simulink model "ConfiguredVirtualVehicleModel"  (R2025b)
settings: Solver=ode14x  StartTime=0  StopTime=inf  FixedStep=.001  RelTol=1e-2  EnableMultiTasking=on
StopFcn:
  | %toc
undefined symbols (not defined in the file or in its folder): CtrlTcuInitGear, DriverPreviewDist, EnvAbsPrs, EnvAirTemp, EnvGrvty, EnvNomFrictionScaling, EnvNominalGrade, EnvWindVelX, EnvWindVelY, EnvWindVelZ, MotoFrmInert, MotoFrmLngth, MotoFrmMass, MotoLowrFrntFrkMass, MotoRearArmLngth, MotoRearArmMass, MotoUpprFrntFrkMass, PlntEngTqMax, RiderMass, Sim3dSensor, trackData
libraries: sm_lib x12, simulink x11, nesl_utility x8, sim3dgroundtruthsensorlib x2, autolibshared x2, vehdynlibdriver x2, instrumentseriallib x2, sharedtransform x1, vehdynlibviscommon x1, autolibutils x1, vehdynlibscenariocommon x1, vehdynlibsteering x1
(part 1 of 5)
settings Model: DataDictionary=VirtualMotoTemplate.sldd  ModifiedByFormat=The MathWorks, Inc.  PauseTimes=23.4  Creator=The MathWorks, Inc.  LastModifiedBy=The MathWorks, Inc.
settings SolverCC: ExtrapolationOrder=2.0  NumberNewtonIterations=2.0  DaesscMode=Fast  ZeroCrossAlgorithm=Adaptive  AlgebraicLoopSolver=TrustRegion  AutoInsertRateTranBlk=on  InsertRTBMode=Never (minimum delay)  DecoupledContinuousIntegration=on  MinimalZcImpactIntegration=on  MaxZcPerStep=1.0
settings DataIOCC: DSMLogging=off  ReturnWorkspaceOutputs=off
settings OptimizationCC: ReuseModelBlockBuffer=off
settings DebuggingCC: SignalInfNanChecking=error  ArtificialAlgebraicLoopMsg=none  MaskedZcDiagnostic=none  IgnoredZcDiagnostic=none  UnconnectedInputMsg=warning  UnconnectedOutputMsg=warning  UnconnectedLineMsg=warning  PregeneratedLibrarySubsystemCodeDiagnostic=none  SubsystemReferenceDiagnosticForUnitTest=warning  ArithmeticOperatorsInVariantConditions=warning
settings HardwareCC: UseEmbeddedCoderFeatures=off
settings ModelReferenceCC: EnableRefExpFcnMdlSchedulingChecks=on  ModelReferenceMinAlgLoopOccurrences=on  PropagateSignalLabelsOutOfModel=off
settings SFSimCC: SimUseLocalCustomCode=off
settings RTWCC: RTWUseLocalCustomCode=off  GPUComputeCapability=3.5  DLArmComputeVersion=19.05  LargeConstantGeneration=WriteOnlyDNNConstantsToDataFiles
settings ExplorerConfigSet: SimMechanicsOpenEditorOnUpdate=off  InternalSimMechanicsExplorerSettings="<ExplorerConfiguration><canonicalview>default</canonicalview><AnimationSetting><BasePlaybackSpeed>1.0</BasePlaybackSpeed><PlaybackSpeedFactor>0.5</PlaybackSpeedFactor></AnimationSetting><TilePanel><TileInfo><Tiles Columns=\"1\" Count=\"1\" Rows=\"1\"><Column Weight=\"1\"/><Row Weight=\"1\"/><Tile Height=\"1\" Width=\"1\" X=\"0\" Y=\"0\"/></Tiles></TileInfo><SceneInfo><SceneViewer><BGColor><R>0.60000002384185791</R><G>0.60000002384185791</G><B>0.60000002384185791</B></BGColor><Camera><DoPerspective>on</DoPerspective><Position><X>48.3730560002180638</X><Y>0.69720714407681017</Y><Z>1.00624025938607131</Z></Position><Center><X>47.6181790802191784</X><Y>1.35307362107727269</Y><Z>1.00624025938607131</Z></Center><Up><X>0</X><Y>0</Y><Z>1</Z></Up><ViewLimDist>1</ViewLimDist><YLim>0.466307658154998583</YLim><XLim>1.00155607891196818</XLim></Camera></SceneViewer></SceneInfo></TilePanel><MechEditorPanel><Cameras><Camera><Id>Camera1</Id><Value><Name>InplaneRightSide</Name><NativeCamera><PositionTrackingFeature>Motorcycle_Vehicle.Body_Steer_Suspension_Wheels.Body_Steer_Suspension_Wheels.In_Plane_Model.Chassis_Tires_and_Areo.Chassis_Body_Suspension_and_Steering.CHASSIS.Chassis_body.CPRr.Camera.Right.base.R</PositionTrackingFeature><CenterTrackingFeature>Motorcycle_Vehicle.Body_Steer_Suspension_Wheels.Body_Steer_Suspension_Wheels.In_Plane_Model.Chassis_Tires_and_Areo.Chassis_Body_Suspension_and_Steering.CHASSIS.Chassis_body.CPRr.Camera.Right.target.R</CenterTrackingFeature><UpVectorTrackingFeature>Motorcycle_Vehicle.Body_Steer_Suspension_Wheels.Body_Steer_Suspension_Wheels.In_Plane_Model.Chassis_Tires_and_Areo.Chassis_Body_Suspension_and_Steering.CHASSIS.Chassis_body.CPRr.Camera.Right.target.R</UpVectorTrackingFeature><CenterTrackingOrigin>off</CenterTrackingOrigin><CenterTrackingDirection>-Y</CenterTrackingDirection><UpVectorTrackingDirection>-Z</UpVectorTrackingDirection></NativeCamera></Value></Camera><Camera><Id>Camera2</Id><Value><Name>OutofPlaneRightSide</Name><NativeCamera><PositionTrackingFeature>Motorcycle_Vehicle.Body_Steer_Suspension_Wheels.Body_Steer_Suspension_Wheels.Out_of_Plane_Model.Chassis_Tires_and_Areo.Chassis_Body_Suspension_and_Steering.CHASSIS.Chassis_body.CPRr.Camera.Right.base.R</PositionTrackingFeature><CenterTrackingFeature>Motorcycle_Vehicle.Body_Steer_Suspension_Wheels.Body_Steer_Suspension_Wheels.Out_of_Plane_Model.Chassis_Tires_and_Areo.Chassis_Body_Suspension_and_Steering.CHASSIS.Chassis_body.CPRr.Camera.Right.base.R</CenterTrackingFeature><UpVectorTrackingFeature>Motorcycle_Vehicle.Body_Steer_Suspension_Wheels.Body_Steer_Suspension_Wheels.Out_of_Plane_Model.Chassis_Tires_and_Areo.Chassis_Body_Suspension_and_Steering.CHASSIS.Chassis_body.CPRr.Camera.Right.base.R</UpVectorTrackingFeature><CenterTrackingOrigin>off</CenterTrackingOrigin><CenterTrackingDirection>-Y</CenterTrackingDirection><UpVectorTrackingDirection>-Z</UpVectorTrackingDirection></NativeCamera></Value></Camera></Cameras><GfxPanelCameraMap><MapElement CameraMLId=\"Camera2\" GfxPanelIndex=\"0\"/></GfxPanelCameraMap><VideoCreator><PlaybackSpeedRatio>1.0</PlaybackSpeedRatio><FrameRate>30</FrameRate><VideoFormat>Motion JPEG AVI</VideoFormat><FrameSize>auto</FrameSize></VideoCreator></MechEditorPanel></ExplorerConfiguration>"

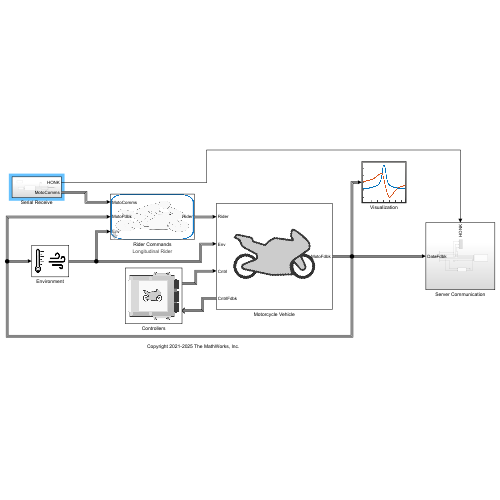
[thumbnail: Simulink's stored preview of the top-level diagram]
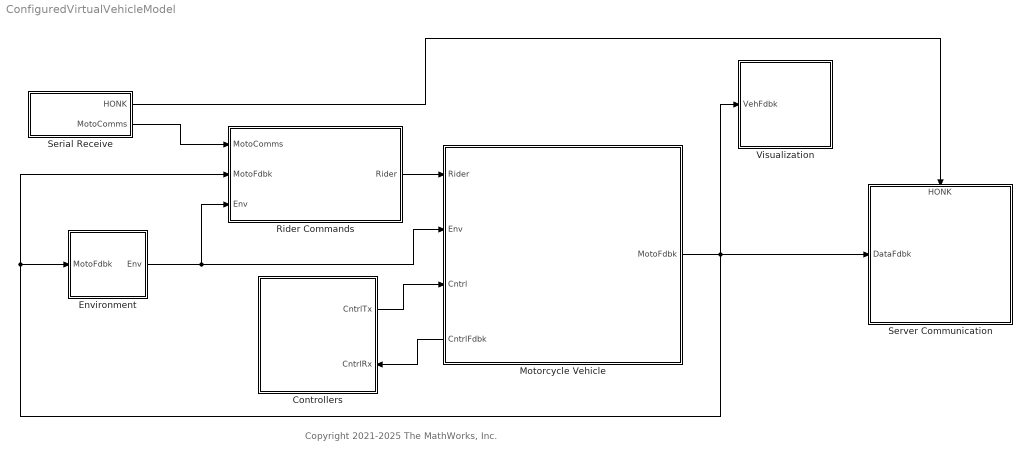
== system ConfiguredVirtualVehicleModel ==
  note: Copyright 2021-2025 The MathWorks, Inc.
  Controllers : Subsystem
      settings: PortSchema="{\"entries\":[{\"content\":{\"sides\":[{\"content\":{},\"type\":\"ConnectorPlacement.EquallySpacedRectSide\",\"uuid\":\"d3abfdf3-59f3-4762-8e4e-957745a11e2c\"},{\"content\":{\"connectorIds\":[\"Out1\",\"In1\"],\"side\":\"RIGHT\"},\"type\":\"ConnectorPlacement.EquallySpacedRectSide\",\"uuid\":\"4c115717-9c17-4631-bd95-1f831e7f83d7\"},{\"content\":{\"side\":\"TOP\"},\"type\":\"ConnectorPlacement.EquallySpacedRectSide\",\"uuid\":\"d2ccb451-5fc1-4147-9a0c-1582624fa182\"}]},\"type\":\"ConnectorPlacement.EquallySpacedConnector\",\"uuid\":\"cab9e2c1-ce8a-4f9c-a024-cef64f8d49c6\"}],\"packageUris\":[\"http://schema.mathworks.com/mf0/Connector/R2020b\"],\"version\":\"1.0\"}"
      mask Display: image('motoECU.png')
  Environment : Subsystem
      mask Display: image('Enviroment.png')
  Motorcycle Vehicle : Subsystem
      settings: PortSchema="{\"entries\":[{\"content\":{\"sides\":[{\"content\":{\"connectorIds\":[\"In1\",\"In2\",\"In3\",\"Out2\"]},\"type\":\"ConnectorPlacement.EquallySpacedRectSide\",\"uuid\":\"175d7041-2aff-4cd5-b9c0-3998d48105ea\"},{\"content\":{\"connectorIds\":[\"Out1\"],\"side\":\"RIGHT\"},\"type\":\"ConnectorPlacement.EquallySpacedRectSide\",\"uuid\":\"0f698ea4-f06f-4552-98b1-af1f0960853e\"},{\"content\":{\"side\":\"TOP\"},\"type\":\"ConnectorPlacement.EquallySpacedRectSide\",\"uuid\":\"8127d405-6a03-4548-a956-3e3bb7246319\"}]},\"type\":\"ConnectorPlacement.EquallySpacedConnector\",\"uuid\":\"b217a386-2802-4b5f-8626-423e606b91b2\"}],\"packageUris\":[\"http://schema.mathworks.com/mf0/Connector/R2020b\"],\"version\":\"1.0\"}"
      mask Display: image('moto.png')
  Rider Commands : Subsystem  VariantControl=0  mask{driverType=Longitudinal Rider, TorqueControlType=No torque control, A=0, D=0.1, I=5, P=150, OutSatLowLmt=-100, OutSatUpLmt=100}
      mask prompts: driverType "Rider type"; TorqueControlType "Torque control"; A "vdynblks:vehdynSteeringSystem:blkPrm_AntiwindGain"; D "vdynblks:vehdynSteeringSystem:blkPrm_DGain"; I "vdynblks:vehdynSteeringSystem:blkPrm_IGain"; P "vdynblks:vehdynSteeringSystem:blkPrm_PGain"; OutSatLowLmt "vdynblks:vehdynSteeringSystem:blkPrm_OutSatLowLmt"; OutSatUpLmt "vdynblks:vehdynSteeringSystem:blkPrm_OutSatUpLmt"
      mask init:
      | [~]=vdynblksdrvrconfig(gcb);
      settings: AttributesFormatString=%<driverType>
      mask Help: eval('vdynblkshelp(''vdmtrrider'')');
      mask TypeOptions driverType: Longitudinal Rider | Open Loop
      mask Callback driverType: [~]=vdynblksdrvrconfig(gcb);
      mask TypeOptions TorqueControlType: Torque PID control | No torque control | Look ahead point model | PID Control
      mask DialogControl A Prompt: Integral anti-windup gain, A []:
      mask DialogControl D Prompt: Derivative gain, D []:
      mask DialogControl I Prompt: Integral gain, I []:
      mask DialogControl P Prompt: Proportional gain, P []:
      mask DialogControl OutSatLowLmt Prompt: Steering torque output saturation lower limit, OutSatLowLmt [Nm]:
      mask DialogControl OutSatUpLmt Prompt: Steering torque output saturation upper limit, OutSatUpLmt [Nm]:
      mask Display: image('rider.png'); % Use "Edit Image" on toolstrip to change.
  Serial Receive : Subsystem
  Server Communication : Subsystem
      settings: PortSchema="{\"entries\":[{\"content\":{\"sides\":[{\"content\":{\"connectorIds\":[\"In1\"]},\"type\":\"ConnectorPlacement.EquallySpacedRectSide\",\"uuid\":\"07e3cf90-2a4b-4b6a-90e3-ec137f6b52d9\"},{\"content\":{\"side\":\"RIGHT\"},\"type\":\"ConnectorPlacement.EquallySpacedRectSide\",\"uuid\":\"79c66d88-e2e2-4982-8f08-c82342e6913b\"},{\"content\":{\"connectorIds\":[\"In2\"],\"side\":\"TOP\"},\"type\":\"ConnectorPlacement.EquallySpacedRectSide\",\"uuid\":\"449d2507-f600-4b7d-af9b-b4af7bc07d5d\"}]},\"type\":\"ConnectorPlacement.EquallySpacedConnector\",\"uuid\":\"5f8e3617-5497-45d3-8aaf-8e2d249ba135\"}],\"packageUris\":[\"http://schema.mathworks.com/mf0/Connector/R2020b\"],\"version\":\"1.0\"}"
  Visualization : Subsystem
      mask Display: image('Visualization.png')
  wires:
  Controllers/1(CntrlTx) -> Motorcycle Vehicle/3(Cntrl)
  Motorcycle Vehicle/2(CntrlFdbk) -> Controllers/1(CntrlRx)
  Environment/1(Env) -> Rider Commands/3(Env), Motorcycle Vehicle/2(Env)
  Motorcycle Vehicle/1(MotoFdbk) -> Server Communication/1(DataFdbk), Rider Commands/2(MotoFdbk), Environment/1(MotoFdbk), Visualization/1(VehFdbk)
  Rider Commands/1(Rider) -> Motorcycle Vehicle/1(Rider)
  Serial Receive/2(MotoComms) -> Rider Commands/1(MotoComms)
  Serial Receive/1(HONK) -> Server Communication/2(HONK)

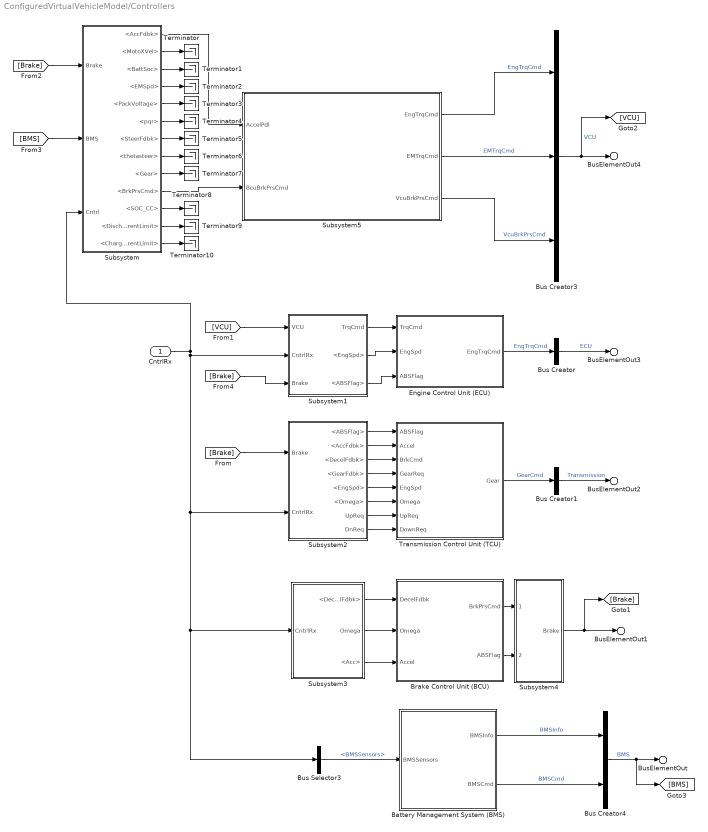
== system ConfiguredVirtualVehicleModel/Controllers ==
  CntrlRx : Inport
  Battery Management System (BMS) : Subsystem  Variant=on  VariantControlMode=label  LabelModeActiveChoice=NoBMS
  Brake Control Unit (BCU) : Subsystem  Variant=on  VariantChoicesSpecifier={'OpenLoopController'}  VariantControlMode=label  LabelModeActiveChoice=OpenLoopController
  Bus Creator : BusCreator  Inputs=1
  Bus Creator1 : BusCreator  Inputs=1
  Bus Creator3 : BusCreator  Inputs=3
  Bus Creator4 : BusCreator  Inputs=2
  Bus Selector3 : BusSelector  OutputSignals=Battery.BMSSensors
  Engine Control Unit (ECU) : Subsystem  Variant=on  VariantChoicesSpecifier={'MotoSimpleECU'}  VariantControlMode=label  LabelModeActiveChoice=MotoSimpleECU
  Subsystem : Subsystem
  Subsystem1 : Subsystem
  Subsystem2 : Subsystem
  Subsystem3 : Subsystem
  Subsystem4 : Subsystem
  Subsystem5 : Subsystem
  Terminator{,1..10} (11 alike) : Terminator
  Transmission Control Unit (TCU) : Subsystem  Variant=on  VariantChoicesSpecifier={'RiderPassThrough'}  VariantControlMode=label  VariantControl=Variant1  LabelModeActiveChoice=RiderPassThrough
  BusElementOut : Outport  PortName=CntrlTx  Element=BMS
  BusElementOut1 : Outport  PortName=CntrlTx  Element=Brake
  BusElementOut2 : Outport  PortName=CntrlTx  Element=Transmission
  BusElementOut3 : Outport  PortName=CntrlTx  Element=ECU
  BusElementOut4 : Outport  PortName=CntrlTx  Element=VCU
  wires:
  Bus Creator/1 -> BusElementOut3/1  "ECU"
  Bus Creator1/1 -> BusElementOut2/1  "Transmission"
  Engine Control Unit (ECU)/1(EngTrqCmd) -> Bus Creator/1  "EngTrqCmd"
  Transmission Control Unit (TCU)/1(" Gear") -> Bus Creator1/1  "GearCmd"
  CntrlRx/1 -> Subsystem1/2(CntrlRx), Subsystem3/1(CntrlRx), Bus Selector3/1, Subsystem2/2(CntrlRx), Subsystem/3(Cntrl)
  Bus Selector3/1 -> Battery Management System (BMS)/1(BMSSensors)  "<BMSSensors>"
  Battery Management System (BMS)/2(BMSCmd) -> Bus Creator4/2  "BMSCmd"
  Bus Creator4/1 -> [BMS], BusElementOut/1  "BMS"
  Battery Management System (BMS)/1(BMSInfo) -> Bus Creator4/1  "BMSInfo"
  Bus Creator3/1 -> [VCU], BusElementOut4/1  "VCU"
  Subsystem5/1(EngTrqCmd) -> Bus Creator3/1  "EngTrqCmd"
  Subsystem5/2(EMTrqCmd) -> Bus Creator3/2  "EMTrqCmd"
  Subsystem5/3(VcuBrkPrsCmd) -> Bus Creator3/3  "VcuBrkPrsCmd"
  [Brake] -> Subsystem/1(Brake)
  [BMS] -> Subsystem/2(BMS)
  Subsystem/1(<AccFdbk>) -> Subsystem5/1(AccelPdl)
  Subsystem/10(<BrkPrsCmd>) -> Subsystem5/2(BcuBrkPrsCmd)
  [Brake] -> Subsystem1/3(Brake)
  Subsystem1/2(<EngSpd>) -> Engine Control Unit (ECU)/2(EngSpd)
  Subsystem1/3(<ABSFlag>) -> Engine Control Unit (ECU)/3(ABSFlag)
  [Brake] -> Subsystem2/1(Brake)
  Subsystem2/1(<ABSFlag>) -> Transmission Control Unit (TCU)/1(ABSFlag)
  Subsystem2/2(<AccFdbk>) -> Transmission Control Unit (TCU)/2(Accel)
  Subsystem2/3(<DecelFdbk>) -> Transmission Control Unit (TCU)/3(BrkCmd)
  Subsystem2/4(<GearFdbk>) -> Transmission Control Unit (TCU)/4(GearReq)
  Subsystem2/5(<EngSpd>) -> Transmission Control Unit (TCU)/5(EngSpd)
  Subsystem2/6(<Omega>) -> Transmission Control Unit (TCU)/6(Omega)
  Subsystem3/1(<DecelFdbk>) -> Brake Control Unit (BCU)/1(DecelFdbk)
  Subsystem3/2(Omega) -> Brake Control Unit (BCU)/2(Omega)
  Subsystem3/3(<Acc>) -> Brake Control Unit (BCU)/3(Accel)
  Subsystem2/7(UpReq) -> Transmission Control Unit (TCU)/7(UpReq)
  Subsystem2/8(DnReq) -> Transmission Control Unit (TCU)/8(DownReq)
  Subsystem4/1(Brake) -> [Brake], BusElementOut1/1
  Brake Control Unit (BCU)/1(BrkPrsCmd) -> Subsystem4/1(BrkPrsCmd)
  Brake Control Unit (BCU)/2(ABSFlag) -> Subsystem4/2(ABSFlag)
  Subsystem/2(<MotoXVel>) -> Terminator/1
  Subsystem/3(<BattSoc>) -> Terminator1/1
  Subsystem/4(<EMSpd>) -> Terminator2/1
  Subsystem/5(<PackVoltage>) -> Terminator3/1
  Subsystem/6(<pqr>) -> Terminator4/1
  Subsystem/7(<SteerFdbk>) -> Terminator5/1
  Subsystem/8(<thetasteer>) -> Terminator6/1
  Subsystem/9(<Gear>) -> Terminator7/1
  Subsystem/11(<SOC_CC>) -> Terminator8/1
  Subsystem/12(<DischargeCurrentLimit>) -> Terminator9/1
  Subsystem/13(<ChargeCurrentLimit>) -> Terminator10/1
  [VCU] -> Subsystem1/1(VCU)
  Subsystem1/1(TrqCmd) -> Engine Control Unit (ECU)/1(TrqCmd)

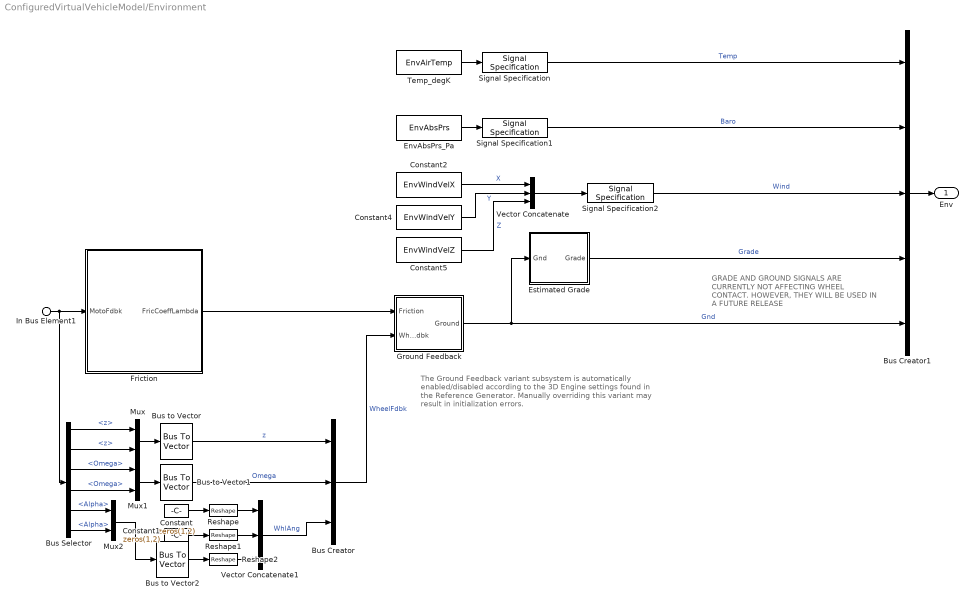
== system ConfiguredVirtualVehicleModel/Environment ==
  note: GRADE AND GROUND SIGNALS ARE CURRENTLY NOT AFFECTING WHEEL CONTACT. HOWEVER, THEY WILL BE USED IN A FUTURE RELEASE
  note: The Ground Feedback variant subsystem is automatically enabled/disabled according to the 3D Engine settings found in the Reference Generator.
      | Manually overriding this variant may result in initialization errors.
  In Bus Element1 : Inport  PortName=MotoFdbk
  Bus Creator : BusCreator  Inputs=3
  Bus Creator1 : BusCreator  Inputs=5
  Bus Selector : BusSelector  OutputSignals=Whl.Genrl.Frnt.Cp.Disp.z,Whl.Genrl.Rear.Cp.Disp.z,Wheels.FrontTire.Omega,Wheels.RearTire.Omega,Wheels.FrontTire.Alpha,Wheels.RearTire.Alpha
  Bus to Vector : BusToVector
  Bus to Vector1 : BusToVector
  Bus to Vector2 : BusToVector
  Constant : Constant  Value=zeros(1,2)
  Constant1 : Constant  Value=zeros(1,2)
  Constant2 : Constant  Value=EnvWindVelX  SampleTime=0
  Constant4 : Constant  Value=EnvWindVelY  SampleTime=0
  Constant5 : Constant  Value=EnvWindVelZ  SampleTime=0
  EnvAbsPrs_Pa : Constant  Value=EnvAbsPrs  SampleTime=0
  Estimated Grade : Subsystem
  Friction : Subsystem  Variant=on  VariantControlMode=label  VariantControl=Choice  LabelModeActiveChoice=Constant Friction
  Ground Feedback : Subsystem  Variant=on  VariantControlMode=label  LabelModeActiveChoice=0
  Mux : Mux  Inputs=2
  Mux1 : Mux  Inputs=2
  Mux2 : Mux  Inputs=2
  Reshape : Reshape  OutputDimensionality=Row vector (2-D)
  Reshape1 : Reshape  OutputDimensionality=Row vector (2-D)
  Reshape2 : Reshape  OutputDimensionality=Row vector (2-D)
  Signal Specification : SignalSpecification  Unit=K
  Signal Specification1 : SignalSpecification  Unit=Pa
  Signal Specification2 : SignalSpecification  Unit=m/s
  Temp_degK : Constant  Value=EnvAirTemp  SampleTime=0
  Vector Concatenate : Concatenate  NumInputs=3
  Vector Concatenate1 : Concatenate  NumInputs=3  Mode=Multidimensional array
  Env : Outport  VectorParamsAs1DForOutWhenUnconnected=off
  wires:
  Constant5/1 -> Vector Concatenate/3  "Z"
  Signal Specification2/1 -> Bus Creator1/3  "Wind"
  Constant4/1 -> Vector Concatenate/2  "Y"
  Ground Feedback/1(Ground) -> Bus Creator1/5, Estimated Grade/1(Gnd)  "Gnd"
  Bus Creator1/1 -> Env/1
  Signal Specification/1 -> Bus Creator1/1  "Temp"
  Signal Specification1/1 -> Bus Creator1/2  "Baro"
  Friction/1(FricCoeffLambda) -> Ground Feedback/1(Friction)
  Estimated Grade/1(Grade) -> Bus Creator1/4  "Grade"
  In Bus Element1/1 -> Friction/1(MotoFdbk), Bus Selector/1
  Bus Selector/2 -> Mux/2  "<z>"
  Bus Selector/1 -> Mux/1  "<z>"
  Mux/1 -> Bus to Vector/1
  Bus to Vector/1 -> Bus Creator/1  "z"
  Bus Selector/3 -> Mux1/1  "<Omega>"
  Bus Selector/4 -> Mux1/2  "<Omega>"
  Mux1/1 -> Bus to Vector1/1
  Bus to Vector1/1 -> Bus Creator/2  "Omega"
  Bus Selector/5 -> Mux2/1  "<Alpha>"
  Bus Selector/6 -> Mux2/2  "<Alpha>"
  Mux2/1 -> Bus to Vector2/1
  Constant/1 -> Reshape/1
  Constant1/1 -> Reshape1/1
  Bus to Vector2/1 -> Reshape2/1
  Reshape/1 -> Vector Concatenate1/1
  Reshape1/1 -> Vector Concatenate1/2
  Reshape2/1 -> Vector Concatenate1/3
  Vector Concatenate1/1 -> Bus Creator/3  "WhlAng"
  Bus Creator/1 -> Ground Feedback/2(WheelFdbk)  "WheelFdbk"
  Constant2/1 -> Vector Concatenate/1  "X"
  Temp_degK/1 -> Signal Specification/1
  EnvAbsPrs_Pa/1 -> Signal Specification1/1
  Vector Concatenate/1 -> Signal Specification2/1

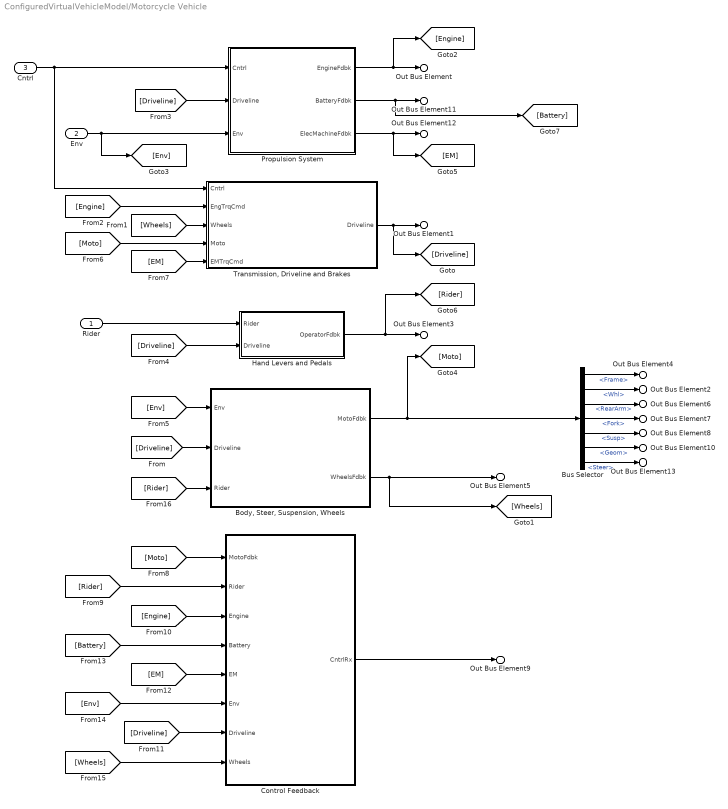
== system ConfiguredVirtualVehicleModel/Motorcycle Vehicle ==
  Rider : Inport
  Env : Inport  Port=2
  Cntrl : Inport  Port=3
  "Body, Steer, Suspension, Wheels" : Subsystem
      mask Display: image('$imagefile'); % Use "Edit Image" on toolstrip to change.
  Bus Selector : BusSelector  OutputSignals=Frame,Whl,RearArm,Fork,Susp,Geom,Steer
  Control Feedback : Subsystem
  Hand Levers and Pedals : Subsystem
  Propulsion System : Subsystem
      mask Display: image('$imagefile'); % Use "Edit Image" on toolstrip to change.
  "Transmission, Driveline and Brakes" : Subsystem
      mask Display: image('$imagefile'); % Use "Edit Image" on toolstrip to change.
  Out Bus Element : Outport  PortName=MotoFdbk  Element=Engine
  Out Bus Element3 : Outport  PortName=MotoFdbk  Element=Rider
  Out Bus Element4 : Outport  PortName=MotoFdbk  Element=Body
  Out Bus Element5 : Outport  PortName=MotoFdbk  Element=Wheels
  Out Bus Element1 : Outport  PortName=MotoFdbk  Element=Driveline
  Out Bus Element2 : Outport  PortName=MotoFdbk  Element=Whl
  Out Bus Element6 : Outport  PortName=MotoFdbk  Element=RearArm
  Out Bus Element7 : Outport  PortName=MotoFdbk  Element=Fork
  Out Bus Element8 : Outport  PortName=MotoFdbk  Element=Susp
  Out Bus Element10 : Outport  PortName=MotoFdbk  Element=Geom
  Out Bus Element11 : Outport  PortName=MotoFdbk  Element=Battery
  Out Bus Element12 : Outport  PortName=MotoFdbk  Element=ElecMachine
  Out Bus Element13 : Outport  PortName=MotoFdbk  Element=Steer
  Out Bus Element9 : Outport  Port=2  PortName=CntrlFdbk
  wires:
  Bus Selector/1 -> Out Bus Element4/1  "<Frame>"
  Bus Selector/2 -> Out Bus Element2/1  "<Whl>"
  Bus Selector/3 -> Out Bus Element6/1  "<RearArm>"
  Bus Selector/4 -> Out Bus Element7/1  "<Fork>"
  Bus Selector/5 -> Out Bus Element8/1  "<Susp>"
  Bus Selector/6 -> Out Bus Element10/1  "<Geom>"
  Propulsion System/1(EngineFdbk) -> [Engine], Out Bus Element/1
  [Driveline] -> Propulsion System/2(Driveline)
  "Transmission, Driveline and Brakes"/1(Driveline) -> [Driveline], Out Bus Element1/1
  [Engine] -> "Transmission, Driveline and Brakes"/2(EngTrqCmd)
  [Wheels] -> "Transmission, Driveline and Brakes"/3(Wheels)
  [Moto] -> "Transmission, Driveline and Brakes"/4(Moto)
  Propulsion System/2(BatteryFdbk) -> [Battery], Out Bus Element11/1
  Propulsion System/3(ElecMachineFdbk) -> Out Bus Element12/1, [EM]
  Rider/1 -> Hand Levers and Pedals/1(Rider)
  [Driveline] -> Hand Levers and Pedals/2(Driveline)
  Hand Levers and Pedals/1(OperatorFdbk) -> [Rider], Out Bus Element3/1
  "Body, Steer, Suspension, Wheels"/1(MotoFdbk) -> Bus Selector/1, [Moto]
  "Body, Steer, Suspension, Wheels"/2(WheelsFdbk) -> [Wheels], Out Bus Element5/1
  [Driveline] -> "Body, Steer, Suspension, Wheels"/2(Driveline)
  Env/1 -> [Env], Propulsion System/3(Env)
  [Env] -> "Body, Steer, Suspension, Wheels"/1(Env)
  [EM] -> "Transmission, Driveline and Brakes"/5(EMTrqCmd)
  Cntrl/1 -> "Transmission, Driveline and Brakes"/1(Cntrl), Propulsion System/1(Cntrl)
  Control Feedback/1(CntrlRx) -> Out Bus Element9/1
  [Moto] -> Control Feedback/1(MotoFdbk)
  [Rider] -> Control Feedback/2(Rider)
  [Engine] -> Control Feedback/3(Engine)
  [EM] -> Control Feedback/5(EM)
  [Battery] -> Control Feedback/4(Battery)
  [Driveline] -> Control Feedback/7(Driveline)
  [Env] -> Control Feedback/6(Env)
  [Wheels] -> Control Feedback/8(Wheels)
  [Rider] -> "Body, Steer, Suspension, Wheels"/3(Rider)
  Bus Selector/7 -> Out Bus Element13/1  "<Steer>"

== system ConfiguredVirtualVehicleModel/Rider Commands ==
  MotoComms : Inport
  MotoFdbk : Inport  Port=2
  Env : Inport  Port=3
  GearGround : Ground
  Rider Commands : Subsystem  Variant=on  VariantControl=Variant1
  Torque Control : Subsystem  Variant=on
  Rider : Outport  VectorParamsAs1DForOutWhenUnconnected=off
  wires:
  MotoComms/1 -> Torque Control/1(MotoRef), Rider Commands/1(MotoComms)
  MotoFdbk/1 -> Torque Control/2(MotoFdbk), Rider Commands/2(MotoFdbk)
  Rider Commands/1(" Rider") -> Torque Control/3(RiderInput)
  Env/1 -> Rider Commands/3(Env)
  Torque Control/1(Rider) -> Rider/1
  GearGround/1 -> Rider Commands/4(GearCmd)

== system ConfiguredVirtualVehicleModel/Serial Receive ==
  Bus Creator : BusCreator  Inputs=3
  Decode : MATLAB Function  TreatAsAtomicUnit=on
  RT : RateTransition  Deterministic=off  OutPortSampleTime=0.001
  Scope : Scope
      settings: ActiveDisplayYMinimum=0.59365579475349917  ActiveDisplayYMaximum=0.83764180505363828  DataLoggingVariableName=ScopeData3
  Serial Configuration : instrumentseriallib/Serial Configuration  Priority=-200000  PortSel=COM6  Port=COM6  ComPort=COM6  BaudRate=115200  DataBits=8  Parity=none  StopBits=1  ByteOrder=little-endian  FlowControl=none  Timeout=10  SimulateUsing=Interpreted execution  BlockInModel=on  aMode=1
  Serial Receive : instrumentseriallib/Serial Receive  Priority=1  PortSel=COM6  Port=COM6  ComPort=COM6  DataType=uint8  SaveDataType=uint8  ToggleHeader=off  Header=[]  ToggleDataSize=on  DataSize=[1 1]  ToggleTerminator=off  Terminator=<none>  CustomTerminator=[]  InputFormat=Column major  EnableBlockingMode=on  ActionDataUnavailable=Output last received value  ActionWhenDataUnavailable=Output last received value  CustomValue=0  SampleTime=0.01  SimulateUsing=Interpreted execution  BlockInModel=on  aMode=1  LibraryInUse=instrumentlib
  HONK : Outport
  MotoComms : Outport  Port=2
  wires:
  Serial Receive/1 -> Decode/1(rawByte)
  Bus Creator/1 -> MotoComms/1  "MotoComms"
  RT/1 -> HONK/1
  Decode/1(Accel) -> Scope/1, Bus Creator/1  "Accel"
  Decode/2(Decel) -> Bus Creator/2  "Decel"
  Decode/3(Gear) -> Bus Creator/3  "Gear"
  Decode/4(HONK) -> RT/1  "Decel"

== system ConfiguredVirtualVehicleModel/Server Communication ==
  DataFdbk : Inport
  HONK : Inport  Port=2
  Bus Selector : BusSelector  OutputSignals=Wheels.RearTire.Omega,Engine.EngineInfo.ExhManGasTemp,Engine.EngineInfo.EoCO2,Engine.EngineInfo.EngSpd,Engine.EngineInfo.FuelVolFlw,Body.BdyFrm.Cg.Vel.xdot
  Performance Calculations : Subsystem
  "Steer, Velocity, Lat Accel" : Scope  NumInputPorts=3
      settings: ActiveDisplayYMinimum=-569.38084213892614  ActiveDisplayYMaximum=94.564320801759081  DataLoggingVariableName=ScopeData2
  Terminator1 : Terminator
  UDPSend : MATLAB Function  TreatAsAtomicUnit=on
  wires:
  DataFdbk/1 -> Bus Selector/1
  Bus Selector/1 -> "Steer, Velocity, Lat Accel"/1, UDPSend/2(angspeed)  "<Omega>"
  Bus Selector/2 -> UDPSend/3(temp), "Steer, Velocity, Lat Accel"/3  "<ExhManGasTemp>"
  Bus Selector/3 -> UDPSend/4(emissions)  "<EoCO2>"
  Bus Selector/4 -> "Steer, Velocity, Lat Accel"/2, UDPSend/1(engspeed)  "<EngSpd>"
  HONK/1 -> UDPSend/6(HONK)
  Performance Calculations/1(US MPG) -> Terminator1/1
  Bus Selector/6 -> Performance Calculations/1(VehSpd)  "<xdot>"
  Bus Selector/5 -> Performance Calculations/2(FuelVolFlow)  "<FuelVolFlw>"
  Performance Calculations/2(L/100Km) -> UDPSend/5(fuel)

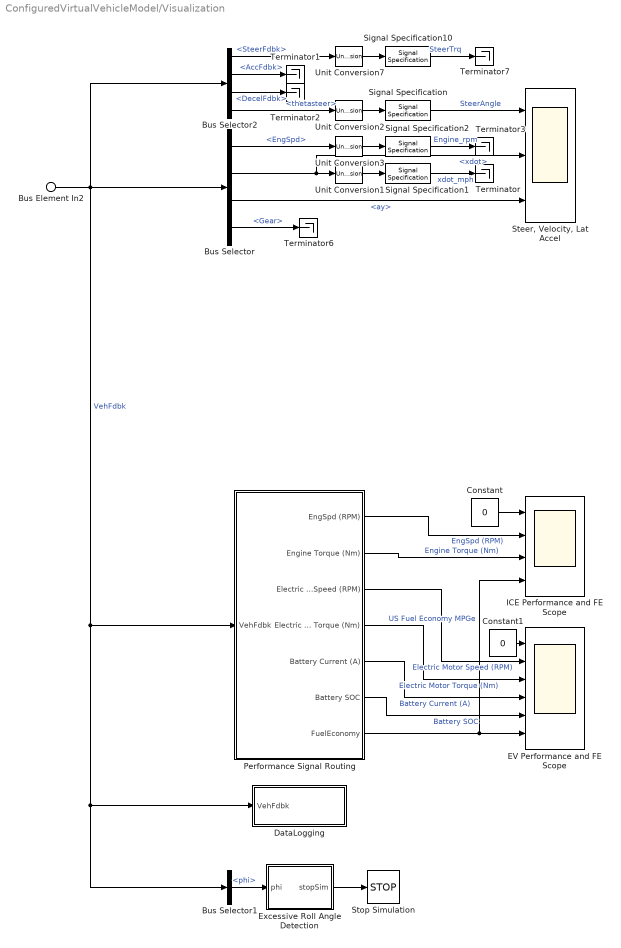
== system ConfiguredVirtualVehicleModel/Visualization ==
  Bus Element In2 : Inport  PortName=VehFdbk
  Bus Selector : BusSelector  OutputSignals=Driveline.EngSpd,Body.BdyFrm.Cg.Vel.xdot,Body.BdyFrm.Cg.Acc.ay,Driveline.Gear
  Bus Selector1 : BusSelector  OutputSignals=Body.InertFrm.Cg.Ang.phi
  Bus Selector2 : BusSelector  OutputSignals=Rider.SteerFdbk,Rider.AccFdbk,Rider.DecelFdbk,Steer.Genrl.Ang.thetasteer
  Constant : Constant  Value=0
  Constant1 : Constant  Value=0
  DataLogging : Subsystem
  EV Performance and FE Scope : Scope  NumInputPorts=6
      settings: SampleTime=0.1  ActiveDisplayYMinimum=-0.55336  ActiveDisplayYMaximum=25.23635
  Excessive Roll Angle Detection : MATLAB Function  TreatAsAtomicUnit=on  SystemSampleTime=.1
  ICE Performance and FE Scope : Scope  NumInputPorts=4
      settings: SampleTime=0.1  ActiveDisplayYMinimum=-3.00968  ActiveDisplayYMaximum=25.77885
  Performance Signal Routing : Subsystem
  Signal Specification : SignalSpecification  Unit=deg
  Signal Specification1 : SignalSpecification  Unit=mph
  Signal Specification10 : SignalSpecification  Unit=N*m
  Signal Specification2 : SignalSpecification  Unit=rpm
  "Steer, Velocity, Lat Accel" : Scope  NumInputPorts=3
      settings: ActiveDisplayYMinimum=-4.93239  ActiveDisplayYMaximum=44.39148
  Stop Simulation : Stop
  Terminator{,1..3,6..7} (6 alike) : Terminator
  Unit Conversion{1..3,7} (4 alike) : UnitConversion
  wires:
  Signal Specification/1 -> "Steer, Velocity, Lat Accel"/1  "SteerAngle"
  Unit Conversion2/1 -> Signal Specification/1
  Bus Selector/3 -> "Steer, Velocity, Lat Accel"/3  "<ay>"
  Bus Element In2/1 -> Bus Selector1/1, DataLogging/1(VehFdbk), Performance Signal Routing/1(VehFdbk), Bus Selector2/1, Bus Selector/1  "VehFdbk"
  Bus Selector/2 -> Unit Conversion1/1, "Steer, Velocity, Lat Accel"/2  "<xdot>"
  Bus Selector2/2 -> Terminator1/1  "<AccFdbk>"
  Bus Selector2/3 -> Terminator2/1  "<DecelFdbk>"
  Bus Selector2/4 -> Unit Conversion2/1  "<thetasteer>"
  Unit Conversion1/1 -> Signal Specification1/1
  Unit Conversion3/1 -> Signal Specification2/1
  Bus Selector/1 -> Unit Conversion3/1  "<EngSpd>"
  Signal Specification2/1 -> Terminator3/1  "Engine_rpm"
  Signal Specification1/1 -> Terminator/1  "xdot_mph"
  Bus Selector/4 -> Terminator6/1  "<Gear>"
  Bus Selector2/1 -> Unit Conversion7/1  "<SteerFdbk>"
  Signal Specification10/1 -> Terminator7/1  "SteerTrq"
  Unit Conversion7/1 -> Signal Specification10/1
  Performance Signal Routing/7(FuelEconomy) -> ICE Performance and FE Scope/4, EV Performance and FE Scope/6  "US Fuel Economy MPGe"
  Performance Signal Routing/1(EngSpd (RPM)) -> ICE Performance and FE Scope/2  "EngSpd (RPM)"
  Performance Signal Routing/2(Engine Torque (Nm)) -> ICE Performance and FE Scope/3  "Engine Torque (Nm)"
  Performance Signal Routing/3(Electric Motor Speed (RPM)) -> EV Performance and FE Scope/2  "Electric Motor Speed (RPM)"
  Performance Signal Routing/4(Electric Motor Torque (Nm)) -> EV Performance and FE Scope/3  "Electric Motor Torque (Nm)"
  Performance Signal Routing/5(Battery Current (A)) -> EV Performance and FE Scope/4  "Battery Current (A)"
  Performance Signal Routing/6(Battery SOC) -> EV Performance and FE Scope/5  "Battery SOC"
  Bus Selector1/1 -> Excessive Roll Angle Detection/1(phi)  "<phi>"
  Excessive Roll Angle Detection/1(stopSim) -> Stop Simulation/1
  Constant/1 -> ICE Performance and FE Scope/1
  Constant1/1 -> EV Performance and FE Scope/1

== system ConfiguredVirtualVehicleModel/Controllers/Battery Management System (BMS) ==
  note: 1) Add Subsystem or Model blocks as valid variant choices.
      | 2) You cannot connect blocks at this level. At simulation, connectivity is automatically
      | determined, based on the active variant and port name matching.
  BMSSensors : Inport
  BMSController : ModelReference  ModelNameDialog=BMSController.slx  SimulationMode=Normal  VariantControl=BMSController  ModelReferenceVersion=11.0
  NoBMS : Subsystem  VariantControl=NoBMS  ReferencedSubsystem=NoBMS
  BMSInfo : Outport
  BMSCmd : Outport  Port=2

== system ConfiguredVirtualVehicleModel/Controllers/Brake Control Unit (BCU) ==
  note: 1) Add Subsystem or Model blocks as valid variant choices.
      | 2) You cannot connect blocks at this level. At simulation, connectivity is automatically
      | determined, based on the active variant and port name matching.
  DecelFdbk : Inport  PortDimensions=2
  Omega : Inport  Port=2
  Accel : Inport  Port=3
  OpenLoopController : ModelReference  ModelNameDialog=OpenLoopController  SimulationMode=Normal  VariantControl=OpenLoopController  ModelReferenceVersion=7.2
  BrkPrsCmd : Outport  VectorParamsAs1DForOutWhenUnconnected=off
  ABSFlag : Outport  Port=2  VectorParamsAs1DForOutWhenUnconnected=off

== system ConfiguredVirtualVehicleModel/Controllers/Engine Control Unit (ECU) ==
  note: 1) Add Subsystem or Model blocks as valid variant choices.
      | 2) You cannot connect blocks at this level. At simulation, connectivity is automatically
      | determined, based on the active variant and port name matching.
  TrqCmd : Inport
  EngSpd : Inport  Port=2
  ABSFlag : Inport  Port=3
  MotoSimpleECU : Subsystem  VariantControl=MotoSimpleECU  ReferencedSubsystem=MotoSimpleECU
  EngTrqCmd : Outport

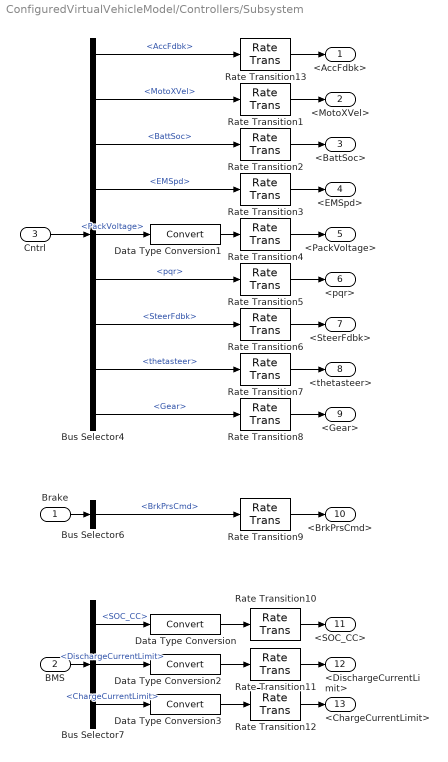
== system ConfiguredVirtualVehicleModel/Controllers/Subsystem ==
  Brake : Inport
  BMS : Inport  Port=2
  Cntrl : Inport  Port=3
  Bus Selector4 : BusSelector  OutputSignals=Rider.AccFdbk,MotoXVel,Battery.BattSoc,Trans.EMSpd,Battery.BMSSensors.PackVoltage,IMU.pqr,Rider.SteerFdbk,Steering.Genrl.Ang.thetasteer,Trans.Gear
  Bus Selector6 : BusSelector  OutputSignals=BrkPrsCmd
  Bus Selector7 : BusSelector  OutputSignals=BMSInfo.SOC.SOC_CC,BMSCmd.CurrentLimitsBus.DischargeCurrentLimit,BMSCmd.CurrentLimitsBus.ChargeCurrentLimit
  Data Type Conversion{,1..3} (4 alike) : DataTypeConversion  SaturateOnIntegerOverflow=off  RndMeth=Floor
  Rate Transition{1..12} (12 alike) : RateTransition  Deterministic=off
  Rate Transition13 : RateTransition  Deterministic=off  OutPortSampleTime=0.001
  <AccFdbk> : Outport
  <MotoXVel> : Outport  Port=2
  <BattSoc> : Outport  Port=3
  <EMSpd> : Outport  Port=4
  <PackVoltage> : Outport  Port=5
  <pqr> : Outport  Port=6
  <SteerFdbk> : Outport  Port=7
  <thetasteer> : Outport  Port=8
  <Gear> : Outport  Port=9
  <BrkPrsCmd> : Outport  Port=10
  <SOC_CC> : Outport  Port=11
  <DischargeCurrentLimit> : Outport  Port=12
  <ChargeCurrentLimit> : Outport  Port=13
  wires:
  Bus Selector4/3 -> Rate Transition2/1  "<BattSoc>"
  Cntrl/1 -> Bus Selector4/1
  Bus Selector4/2 -> Rate Transition1/1  "<MotoXVel>"
  Bus Selector4/6 -> Rate Transition5/1  "<pqr>"
  Bus Selector7/1 -> Data Type Conversion/1  "<SOC_CC>"
  Bus Selector7/2 -> Data Type Conversion2/1  "<DischargeCurrentLimit>"
  Bus Selector4/8 -> Rate Transition7/1  "<thetasteer>"
  Bus Selector4/1 -> Rate Transition13/1  "<AccFdbk>"
  BMS/1 -> Bus Selector7/1
  Bus Selector7/3 -> Data Type Conversion3/1  "<ChargeCurrentLimit>"
  Bus Selector4/4 -> Rate Transition3/1  "<EMSpd>"
  Brake/1 -> Bus Selector6/1
  Bus Selector4/9 -> Rate Transition8/1  "<Gear>"
  Bus Selector4/7 -> Rate Transition6/1  "<SteerFdbk>"
  Bus Selector6/1 -> Rate Transition9/1  "<BrkPrsCmd>"
  Bus Selector4/5 -> Data Type Conversion1/1  "<PackVoltage>"
  Data Type Conversion1/1 -> Rate Transition4/1
  Data Type Conversion/1 -> Rate Transition10/1
  Data Type Conversion2/1 -> Rate Transition11/1
  Data Type Conversion3/1 -> Rate Transition12/1
  Rate Transition1/1 -> <MotoXVel>/1
  Rate Transition2/1 -> <BattSoc>/1
  Rate Transition3/1 -> <EMSpd>/1
  Rate Transition4/1 -> <PackVoltage>/1
  Rate Transition5/1 -> <pqr>/1
  Rate Transition6/1 -> <SteerFdbk>/1
  Rate Transition7/1 -> <thetasteer>/1
  Rate Transition8/1 -> <Gear>/1
  Rate Transition9/1 -> <BrkPrsCmd>/1
  Rate Transition10/1 -> <SOC_CC>/1
  Rate Transition11/1 -> <DischargeCurrentLimit>/1
  Rate Transition12/1 -> <ChargeCurrentLimit>/1
  Rate Transition13/1 -> <AccFdbk>/1

== system ConfiguredVirtualVehicleModel/Controllers/Subsystem1 ==
  VCU : Inport
  CntrlRx : Inport  Port=2
  Brake : Inport  Port=3
  Bus Selector2 : BusSelector  OutputSignals=Engine.EngineInfo.EngSpd
  Bus Selector4 : BusSelector  OutputSignals=EngTrqCmd
  Bus Selector6 : BusSelector  OutputSignals=ABSFlag
  Rate Transition1 : RateTransition  Deterministic=off
  Rate Transition2 : RateTransition  Deterministic=off
  Rate Transition3 : RateTransition  Deterministic=off
  TrqCmd : Outport
  <EngSpd> : Outport  Port=2
  <ABSFlag> : Outport  Port=3
  wires:
  Bus Selector2/1 -> Rate Transition2/1  "<EngSpd>"
  Bus Selector6/1 -> Rate Transition1/1  "<ABSFlag>"
  Brake/1 -> Bus Selector6/1
  CntrlRx/1 -> Bus Selector2/1
  Rate Transition1/1 -> <ABSFlag>/1
  Rate Transition2/1 -> <EngSpd>/1
  VCU/1 -> Bus Selector4/1
  Bus Selector4/1 -> Rate Transition3/1  "<EngTrqCmd>"
  Rate Transition3/1 -> TrqCmd/1

== system ConfiguredVirtualVehicleModel/Controllers/Subsystem2 ==
  Brake : Inport
  CntrlRx : Inport  Port=2
  Bus Selector1 : BusSelector  OutputSignals=Rider.AccFdbk,Rider.DecelFdbk,Rider.GearFdbk,Engine.EngineInfo.EngSpd,Wheels.FrontTire.Omega,Wheels.RearTire.Omega
  Bus Selector5 : BusSelector  OutputSignals=ABSFlag
  Ground : Ground
  Ground1 : Ground
  Mux : Mux  Inputs=2
  Rate Transition{1..4,6..8} (7 alike) : RateTransition  Deterministic=off
  Rate Transition5 : RateTransition  Commented=through  Deterministic=off
  Signal Specification : SignalSpecification  Commented=through  Unit=rpm
  Unit Conversion : UnitConversion
  <ABSFlag> : Outport
  <AccFdbk> : Outport  Port=2
  <DecelFdbk> : Outport  Port=3
  <GearFdbk> : Outport  Port=4
  <EngSpd> : Outport  Port=5
  <Omega> : Outport  Port=6
  UpReq : Outport  Port=7
  DnReq : Outport  Port=8
  wires:
  Bus Selector1/6 -> Mux/2  "<Omega>"
  Brake/1 -> Bus Selector5/1
  Bus Selector1/4 -> Unit Conversion/1  "<EngSpd>"
  Bus Selector1/1 -> Rate Transition2/1  "<AccFdbk>"
  Bus Selector1/2 -> Rate Transition3/1  "<DecelFdbk>"
  Bus Selector1/3 -> Rate Transition4/1  "<GearFdbk>"
  CntrlRx/1 -> Bus Selector1/1
  Bus Selector5/1 -> Rate Transition1/1  "<ABSFlag>"
  Rate Transition8/1 -> DnReq/1
  Rate Transition7/1 -> UpReq/1
  Ground1/1 -> Rate Transition8/1
  Ground/1 -> Rate Transition7/1
  Rate Transition1/1 -> <ABSFlag>/1
  Rate Transition2/1 -> <AccFdbk>/1
  Rate Transition3/1 -> <DecelFdbk>/1
  Rate Transition4/1 -> <GearFdbk>/1
  Rate Transition5/1 -> <EngSpd>/1
  Rate Transition6/1 -> <Omega>/1
  Bus Selector1/5 -> Mux/1  "<Omega>"
  Mux/1 -> Rate Transition6/1
  Unit Conversion/1 -> Signal Specification/1
  Signal Specification/1 -> Rate Transition5/1  "EngSpd"

== system ConfiguredVirtualVehicleModel/Controllers/Subsystem3 ==
  CntrlRx : Inport
  Bus Selector : BusSelector  OutputSignals=Rider.DecelFdbk,Wheels.FrontTire.Omega,Wheels.RearTire.Omega,IMU.Acc
  Mux : Mux  Inputs=2
  Rate Transition : RateTransition  Deterministic=off
  Rate Transition1 : RateTransition  Deterministic=off
  Rate Transition2 : RateTransition  Deterministic=off
  Unary Minus : UnaryMinus
  <DecelFdbk> : Outport
  Omega : Outport  Port=2
  <Acc> : Outport  Port=3
  wires:
  Unary Minus/1 -> Rate Transition1/1
  Mux/1 -> Unary Minus/1
  Bus Selector/1 -> Rate Transition/1  "<DecelFdbk>"
  Bus Selector/4 -> Rate Transition2/1  "<Acc>"
  CntrlRx/1 -> Bus Selector/1
  Rate Transition/1 -> <DecelFdbk>/1
  Rate Transition1/1 -> Omega/1
  Rate Transition2/1 -> <Acc>/1
  Bus Selector/3 -> Mux/2  "<Omega>"
  Bus Selector/2 -> Mux/1  "<Omega>"

== system ConfiguredVirtualVehicleModel/Controllers/Subsystem4 ==
  BrkPrsCmd : Inport
  ABSFlag : Inport  Port=2
  Bus Creator2 : BusCreator  Inputs=2
  Data Type Conversion : DataTypeConversion  OutDataTypeStr=double  SaturateOnIntegerOverflow=off  RndMeth=Floor
  Data Type Conversion1 : DataTypeConversion  OutDataTypeStr=boolean  SaturateOnIntegerOverflow=off  RndMeth=Floor
  First Order Hold : FirstOrderHold  ErrorTolerance=0.1  AllowContinuousInput=on
  First Order Hold1 : FirstOrderHold  ErrorTolerance=1  AllowContinuousInput=on
  Brake : Outport
  wires:
  First Order Hold/1 -> Bus Creator2/2  "BrkPrsCmd"
  Data Type Conversion1/1 -> Bus Creator2/1  "ABSFlag"
  Bus Creator2/1 -> Brake/1  "Brake"
  BrkPrsCmd/1 -> First Order Hold/1
  ABSFlag/1 -> Data Type Conversion/1
  Data Type Conversion/1 -> First Order Hold1/1
  First Order Hold1/1 -> Data Type Conversion1/1

== system ConfiguredVirtualVehicleModel/Controllers/Subsystem5 ==
  AccelPdl : Inport
  BcuBrkPrsCmd : Inport  Port=2  SampleTime=0.01
  Acc to Torque Request : Gain  Gain=max(PlntEngTqMax)
  EngTrqCmd : Outport  OutDataTypeStr=double  PortDimensions=1  VectorParamsAs1DForOutWhenUnconnected=off
  EMTrqCmd : Outport  Port=2  VectorParamsAs1DForOutWhenUnconnected=off
  VcuBrkPrsCmd : Outport  Port=3  PortDimensions=2  VectorParamsAs1DForOutWhenUnconnected=off
  wires:
  Acc to Torque Request/1 -> EMTrqCmd/1, EngTrqCmd/1
  BcuBrkPrsCmd/1 -> VcuBrkPrsCmd/1
  AccelPdl/1 -> Acc to Torque Request/1

== system ConfiguredVirtualVehicleModel/Controllers/Transmission Control Unit (TCU) ==
  ABSFlag : Inport  PortDimensions=2
  Accel : Inport  Port=2
  BrkCmd : Inport  Port=3  PortDimensions=2
  GearReq : Inport  Port=4
  EngSpd : Inport  Port=5
  Omega : Inport  Port=6  Unit=rad/s
  UpReq : Inport  Port=7
  DownReq : Inport  Port=8  Unit=rad/s
  RiderPassThrough : ModelReference  ModelNameDialog=RiderPassThrough  SimulationMode=Normal  VariantControl=RiderPassThrough  ModelReferenceVersion=7.0
  " Gear" : Outport  VectorParamsAs1DForOutWhenUnconnected=off

== system ConfiguredVirtualVehicleModel/Environment/Estimated Grade ==
  Gnd : Inport
  Atan : Trigonometry  Operator=atan
  Bus Selector : BusSelector  OutputSignals=z  OutputAsBus=on
  Bus to Vector : BusToVector
  Constant Grade : Constant  Value=EnvNominalGrade  SampleTime=-1
  Constant1 : Constant  Value=MotoFrmLngth  SampleTime=-1
  Divide : Product  Inputs=*/
  Grade Source : ManualSwitch  CurrentSetting=0
  Selector : Selector  InputPortWidth=2  IndexOptions=Index vector (dialog)  Indices=[1]  OutputSizes=1
  Selector1 : Selector  InputPortWidth=2  IndexOptions=Index vector (dialog)  Indices=[2]  OutputSizes=1
  Signal Specification : SignalSpecification  Unit=rad
  Signal Specification1 : SignalSpecification  Unit=deg
  Signal Specification2 : SignalSpecification  Unit=deg
  Subtract : Sum  Inputs=+-
  Unit Conversion : UnitConversion
  Grade : Outport  PortDimensions=1
  wires:
  Divide/1 -> Atan/1
  Bus Selector/1 -> Bus to Vector/1
  Selector/1 -> Subtract/1
  Signal Specification/1 -> Unit Conversion/1
  Constant1/1 -> Divide/2
  Selector1/1 -> Subtract/2
  Subtract/1 -> Divide/1
  Atan/1 -> Signal Specification/1
  Grade Source/1 -> Grade/1  "Grade"
  Gnd/1 -> Bus Selector/1
  Bus to Vector/1 -> Selector1/1, Selector/1
  Constant Grade/1 -> Signal Specification2/1
  Signal Specification2/1 -> Grade Source/2
  Unit Conversion/1 -> Signal Specification1/1
  Signal Specification1/1 -> Grade Source/1  "Grade"

== system ConfiguredVirtualVehicleModel/Environment/Friction ==
  MotoFdbk : Inport
  Constant Friction : Subsystem  VariantControl=Constant Friction
  Varying Friction : Subsystem  VariantControl=Varying Friction
  FricCoeffLambda : Outport

== system ConfiguredVirtualVehicleModel/Environment/Ground Feedback ==
  Friction : Inport
  WheelFdbk : Inport  Port=2
  3D Engine : Subsystem  VariantControl=1
  Constant : Subsystem  VariantControl=0
  Ground : Outport  VectorParamsAs1DForOutWhenUnconnected=off

== system ConfiguredVirtualVehicleModel/Motorcycle Vehicle/Body, Steer, Suspension, Wheels ==
  Env : Inport
  Driveline : Inport  Port=2
  Rider : Inport  Port=3
  "Body, Steer, Suspension, Wheels" : Subsystem  Variant=on  VariantChoicesSpecifier={'In_Plane_ModelArchitecture'}  VariantControlMode=label  VariantControl=Choice  LabelModeActiveChoice=In_Plane_ModelArchitecture
      mask Display: disp('Body,Steer,Suspension,Wheels');
  Chassis Input : Subsystem
  Chassis Output : Subsystem
  MotoFdbk : Outport
  WheelsFdbk : Outport  Port=2
  wires:
  Chassis Input/1(Wind) -> "Body, Steer, Suspension, Wheels"/1(WindXYZ)
  "Body, Steer, Suspension, Wheels"/1(Moto) -> Chassis Output/1(Moto)
  Chassis Input/2(BrkPrs) -> "Body, Steer, Suspension, Wheels"/2(BrkPrs)
  "Body, Steer, Suspension, Wheels"/2(Wheels) -> Chassis Output/2(Wheels)
  Chassis Input/4(MDrvArmR) -> "Body, Steer, Suspension, Wheels"/4(MDrvArmR)
  Chassis Input/6(ScaleFactrs) -> "Body, Steer, Suspension, Wheels"/6(ScaleFactrs)
  Chassis Input/3(MDrvSprtR) -> "Body, Steer, Suspension, Wheels"/3(MDrvSprtR)
  Chassis Input/5(MDrvFrm) -> "Body, Steer, Suspension, Wheels"/5(MDrvFrm)
  Env/1 -> Chassis Input/1(Env)
  Driveline/1 -> Chassis Input/2(Driveline)
  Chassis Output/2(WheelsFdbk) -> WheelsFdbk/1
  Chassis Output/1(MotoFdbk) -> MotoFdbk/1
  Chassis Input/7(SteerCmd) -> "Body, Steer, Suspension, Wheels"/7(SteerCmd)
  Rider/1 -> Chassis Input/3(Rider)

== system ConfiguredVirtualVehicleModel/Motorcycle Vehicle/Control Feedback ==
  MotoFdbk : Inport
  Rider : Inport  Port=2
  Engine : Inport  Port=3
  Battery : Inport  Port=4
  EM : Inport  Port=5
  Env : Inport  Port=6
  Driveline : Inport  Port=7
  Wheels : Inport  Port=8
  Bus Selector1 : BusSelector  OutputSignals=Steer
  Bus Selector2 : BusSelector  OutputSignals=Susp
  Bus Selector7 : BusSelector  OutputSignals=BattSoc,BattVolt,BattCurr,BattPwr,BMSSensors  OutputAsBus=on
  Bus Selector8 : BusSelector  OutputSignals=Frame.BdyFrm.Cg.Vel.xdot  OutputAsBus=on
  Bus Selector9 : BusSelector  OutputSignals=EMTrq,EMPwrElec  OutputAsBus=on
  Variant Subsystem : Subsystem  Variant=on  VariantControlMode=label  LabelModeActiveChoice=No_IMU_Sensor
  Bus Element Out : Outport  PortName=CntrlRx  Element=MotoXVel
  Bus Element Out1 : Outport  PortName=CntrlRx  Element=Rider
  Bus Element Out2 : Outport  PortName=CntrlRx  Element=Engine
  Bus Element Out3 : Outport  PortName=CntrlRx  Element=Trans
  Bus Element Out4 : Outport  PortName=CntrlRx  Element=Battery
  Bus Element Out5 : Outport  PortName=CntrlRx  Element=EM
  Bus Element Out7 : Outport  PortName=CntrlRx  Element=Wheels
  Bus Element Out8 : Outport  PortName=CntrlRx  Element=IMU
  Bus Element Out9 : Outport  PortName=CntrlRx  Element=Env
  Bus Element Out10 : Outport  PortName=CntrlRx  Element=Steering
  Bus Element Out11 : Outport  PortName=CntrlRx  Element=Suspension
  wires:
  Bus Selector2/1 -> Bus Element Out11/1  "<Susp>"
  Wheels/1 -> Bus Element Out7/1
  Bus Selector7/1 -> Bus Element Out4/1  "Battery"
  Bus Selector8/1 -> Bus Element Out/1  "Moto"
  Bus Selector9/1 -> Bus Element Out5/1  "EM"
  Engine/1 -> Bus Element Out2/1
  Battery/1 -> Bus Selector7/1
  EM/1 -> Bus Selector9/1
  MotoFdbk/1 -> Variant Subsystem/1(MotoFdbk), Bus Selector1/1, Bus Selector2/1, Bus Selector8/1  "Moto"
  Variant Subsystem/1(IMU) -> Bus Element Out8/1  "IMU"
  Rider/1 -> Bus Element Out1/1  "Rider"
  Env/1 -> Bus Element Out9/1  "Env"
  Bus Selector1/1 -> Bus Element Out10/1  "<Steer>"
  Driveline/1 -> Bus Element Out3/1

== system ConfiguredVirtualVehicleModel/Motorcycle Vehicle/Hand Levers and Pedals ==
  Rider : Inport
  Driveline : Inport  Port=2
  Hand Levers and Pedals : Subsystem
  Pedal Cluster Input : Subsystem
  Pedal Cluster Output : Subsystem
  OperatorFdbk : Outport
  wires:
  Hand Levers and Pedals/4(GearFdbk) -> Pedal Cluster Output/4(GearFdbk)
  Hand Levers and Pedals/2(AccFdbk) -> Pedal Cluster Output/2(AccFdbk)
  Pedal Cluster Input/5(BrkPrs) -> Hand Levers and Pedals/5(BrkPrs)
  Pedal Cluster Input/1(SteerCmd) -> Hand Levers and Pedals/1(SteerCmd)
  Pedal Cluster Input/6(StrWhlTrq) -> Hand Levers and Pedals/6(StrWhlTrq)
  Pedal Cluster Input/3(DecelCmd) -> Hand Levers and Pedals/3(DecelCmd)
  Hand Levers and Pedals/3(DecelFdbk) -> Pedal Cluster Output/3(DecelFdbk)
  Pedal Cluster Input/2(AccelCmd) -> Hand Levers and Pedals/2(AccCmd)
  Pedal Cluster Input/4(GearCmd) -> Hand Levers and Pedals/4(GearCmd)
  Rider/1 -> Pedal Cluster Input/1(Rider)
  Hand Levers and Pedals/1(SteerFdbk) -> Pedal Cluster Output/1(SteerFdbk)
  Pedal Cluster Output/1(OperatorFdbk) -> OperatorFdbk/1
  Driveline/1 -> Pedal Cluster Input/2(Driveline)

== system ConfiguredVirtualVehicleModel/Motorcycle Vehicle/Propulsion System ==
  Cntrl : Inport
  Driveline : Inport  Port=2
  Env : Inport  Port=3
  Actuators : Subsystem  Variant=on  VariantChoicesSpecifier={'MotoMappedEngine'}  VariantControlMode=label  LabelModeActiveChoice=MotoMappedEngine
  Electrical System Input : Subsystem
  Engine Input : Subsystem
  EngineFdbk : Outport
  BatteryFdbk : Outport  Port=2
  ElecMachineFdbk : Outport  Port=3
  wires:
  Actuators/1(Eng) -> EngineFdbk/1
  Engine Input/2(EngSpd) -> Actuators/2(EngSpd)
  Cntrl/1 -> Electrical System Input/1(Cntrl), Engine Input/1(Cntrl)
  Engine Input/1(EngTrqCmd) -> Actuators/1(TrqCmd)
  Driveline/1 -> Electrical System Input/2(Driveline), Engine Input/2(Driveline)
  Actuators/2(Battery) -> BatteryFdbk/1
  Actuators/3(ElecMachine) -> ElecMachineFdbk/1
  Electrical System Input/1(EMTrqCmd) -> Actuators/3(EMTrqCmd)
  Electrical System Input/2(EMSpd) -> Actuators/4(EMSpd)
  Electrical System Input/3(AmbTemp) -> Actuators/5(AmbTemp)
  Env/1 -> Electrical System Input/3(Env)

== system ConfiguredVirtualVehicleModel/Motorcycle Vehicle/Transmission, Driveline and Brakes ==
  Cntrl : Inport
  EngTrqCmd : Inport  Port=2
  Wheels : Inport  Port=3
  Moto : Inport  Port=4
  EMTrqCmd : Inport  Port=5
  Brake Hydraulics : Subsystem
  Driveline Input : Subsystem
  Driveline Output : Subsystem
  Transmission and Driveline : Subsystem
  Driveline : Outport
  wires:
  Transmission and Driveline/2(Gear) -> Driveline Output/2(Gear)
  Driveline Input/6(MBrkR.) -> Transmission and Driveline/6(MBrkR)
  Driveline Input/3(FCpR.) -> Transmission and Driveline/3(FCpR)
  Transmission and Driveline/1(EngSpd) -> Driveline Output/1(EngSpd)
  Driveline Input/1(EngTrq) -> Transmission and Driveline/1(EngTrq)
  Driveline Input/4(ThetaFrm.) -> Transmission and Driveline/4(ThetaFrm)
  Transmission and Driveline/3(Info) -> Driveline Output/3(Info)
  Driveline Input/2(GearCmd) -> Transmission and Driveline/2(GearCmd)
  Driveline Input/7(AngAWhlR.) -> Transmission and Driveline/7(AngAWhlR)
  Driveline Input/5(ThetaArmR.) -> Transmission and Driveline/5(ThetaArmR)
  Cntrl/1 -> Driveline Input/1(Cntrl)
  EngTrqCmd/1 -> Driveline Input/2(EngTrqCmd)
  Wheels/1 -> Driveline Input/3(Wheels)
  Moto/1 -> Driveline Input/4(Moto)
  Driveline Output/1(Driveline) -> Driveline/1  "Driveline"
  Driveline Input/8(EMTrq) -> Transmission and Driveline/8(EMTrq)
  Transmission and Driveline/4(EMSpd) -> Driveline Output/4(EMSpd)
  EMTrqCmd/1 -> Driveline Input/5(EMTrqCmd)
  Driveline Input/9(BrkPrsCmd) -> Brake Hydraulics/1(BrkPrsCmd)
  Brake Hydraulics/1(BrkPrs) -> Driveline Output/5(BrkPrs)

== system ConfiguredVirtualVehicleModel/Rider Commands/Rider Commands ==
  MotoComms : Inport
  MotoFdbk : Inport  Port=2
  Env : Inport  Port=3
  GearCmd : Inport  Port=4
  Longitudinal Rider : Subsystem  VariantControl=driverType==1
  Open Loop : Subsystem  VariantControl=driverType==2
  Predictive Rider : Subsystem  VariantControl=driverType==4
  Predictive Stanley Rider : Subsystem  VariantControl=driverType==3
  Roll angle control : Subsystem  VariantControl=driverType==6
  Target trajectory following - Look ahead point : Subsystem  VariantControl=driverType==5
  " Rider" : Outport  VectorParamsAs1DForOutWhenUnconnected=off

== system ConfiguredVirtualVehicleModel/Rider Commands/Torque Control ==
  note: 1) Add Subsystem or Model blocks as valid variant choices.
      | 2) You cannot connect blocks at this level. At simulation, connectivity is automatically
      | determined, based on the active variant and port name matching.
  MotoRef : Inport
  MotoFdbk : Inport  Port=2
  RiderInput : Inport  Port=3
  AngleToTorque : Subsystem  VariantControl=TorqueControlType == 1  mask{DbWdth=0.05, StrRng=pi/4}
      mask prompts: DbWdth "Steering deadband width, DbWdth [rad]:"; StrRng "Steering angle limit, StrRng [rad]"
  Look ahead point model : Subsystem  VariantControl=TorqueControlType == 3
  NoTorqueControl : Subsystem  VariantControl=TorqueControlType == 2
  PID Control : Subsystem  VariantControl=TorqueControlType == 4
  Rider : Outport
